simulink model "Main_bikesim2"  (R2024b)
settings: Solver=FixedStepAuto  StartTime=0.0  StopTime=sim_time-0.02  FixedStep=0.005
undefined symbols (not defined in the file): A_d, Ad_t, B_d, Bd_t, bike_model, bike_params, C1, C2, C_t, counter, D1, D2, D_t, e1_max, g, hor_dis, I_balancing_outer, initial_state, initial_state_estimate, k1, k2, Kalman_gain1, Kalman_gain2, linearized_sys, mpc_outer_params, P_balancing_inner, P_balancing_outer, pert_deltadot_state, pert_deltadot_state_fun, pert_phidot_state, pert_phidot_state_fun, Psiref, ref_dis, ref_start_idx, sigbuilder_block, T, Ts, v, Xref, Yref
libraries: simulink x8, slpidlib x2, eeGeneralControl x1
(part 2 of 2)

== matlab function Main_bikesim2/State estimator1/Linearized Bicycle Model on Constant Velocity ==
  data: Est_States input; dot_delta input; y input; Kalman_gain1 input; Kalman_gain2 input; bike_params input; Est_states output; flag input; A_d parameter; B_d parameter; C1 parameter; C2 parameter; D1 parameter; D2 parameter; T parameter
function Est_states  = fcn(Est_States, dot_delta, y, Kalman_gain1, Kalman_gain2, bike_params, flag, A_d, B_d, C1, C2, D1, D2, T)
% description 
% Inputs
%   Est_States := [X Y psi phi phi_dot delta v] are global at time t 
%   dot_delta_e := effective steering rate
%   y := measurement vector
%   Kalman_gain1 := Computed state_feedback gain including GPS meas
%   Kalman_gain2 := Computed state_feedback gain excluding GPS meas
%   bike_params := vector of bike parameters + gravity
%   Ts := Estimator sampling rate
%   v := constant velocity
%   flag := [0-1] increasing counter reseted at 1. When flag == 0 means
%           that GPS measurement is available
%
% Outputs
%   Est_states : = [X Y psi phi phi_dot delta v] global at time t+1


% Transform the states to local frame 
    Est_States_l = zeros(7,1);
    
    Est_States_l(1) = Est_States(1) * cos(Est_States(3)) + Est_States(2) * sin(Est_States(3));
    Est_States_l(2) = -Est_States(1) * sin(Est_States(3)) + Est_States(2) * cos(Est_States(3));
    Est_States_l(3) = 0;        % direction of bike is aligned with X local frame
    Est_States_l(4) = Est_States(4);
    Est_States_l(5) = Est_States(5);
    Est_States_l(6) = Est_States(6);
    Est_States_l(7) = Est_States(7);

% Transform measurements to local frame
    y_l = zeros(size(y));

    y_l(1) = y(1) * cos(Est_States(3)) + y(2) * sin(Est_States(3));
    y_l(2) = -y(1) * sin(Est_States(3)) + y(2) * cos(Est_States(3)); 
    y_l(3) = y(3);
    y_l(4) = y(4);
    y_l(5) = y(5);
    y_l(6) = y(6);
    y_l(7) = y(7);

% Correct for parameter values/sensor positions
% The parameters/positions are measures by us (can differ from true values)
X_gps_mod = bike_params(1);
Y_gps_mod = bike_params(2);
H_gps_mod = bike_params(3);

y_l(1) = y_l(1) - X_gps_mod;
y_l(2) = y_l(2) - Y_gps_mod - H_gps_mod*sin(Est_States(4));

% IMU correction
raw_acc  = [0 y_l(3) 0];
raw_gyro = [y_l(4) 0 y_l(5)];

% Apply the correction to the accelerometer measurement
acc_corr = T*raw_acc';

% Apply the correction to the gyro measurement
gyro_corr = T*raw_gyro';
% Results
y_l(3) =acc_corr(2) ;
y_l(4) =gyro_corr(1) ;
y_l(5) =gyro_corr(3) ;
% 
% % Continuous Time update in local frame TODO: x(t+1) = (I+A delta_T)h_hat(t)
%     states_dot = zeros(7,1);
%     
%     states_dot(1) = Est_States(7);
%     states_dot(2) = v * (Est_States_l(3) + (lr/(lr+lf))*Est_States(6) );
%     states_dot(3) = (v/(lr+lf)) * Est_States(6);
%     states_dot(4) = Est_States(5);
%     states_dot(5) =(g/h)*Est_States(4) + ((lr*v)/((lr+lf)*h))*sin(lambda)*dot_delta + ((h*v^2-g*lr*c)/((lr+lf)*h^2))*sin(lambda)*Est_States(6);
%     states_dot(6) = dot_delta;
%     states_dot(7) = 0;
% 
% % Discrete time update in local 
%     Est_States_l = Est_States_l + states_dot * Ts; 

% % C identity is used to see if the code runs
%     sen = zeros(6,1);
%     sen(1)      = States_l(1);  
%     sen(2)      = States_l(2);
%     %sen(3)      = States_l(3);
%     sen(3)      = States_l(4);
%     sen(4)      = States_l(5);
%     sen(5)      = States_l(6);
%     sen(6)      = States_l(7);

% % Transform measurements into local frame to see if code runs
%     meas_l = zeros(6,1);
%     meas_l(1) = meas(1) * cos(States(3)) + meas(2) * sin(States(3));
%     meas_l(2) = -meas(1) * sin(States(3)) + meas(2) * cos(States(3));
%     meas_l(3) = 0;
%     meas_l(3) = meas(3)-States(3);  
%     meas_l(3) = meas(4);
%     meas_l(4) = meas(5);
%     meas_l(5) = meas(6);
%     meas_l(6) = meas(7);
%     meas_l(7) = meas(7);

% Time update in local frame (from t to t+1)

    % Time update
     Est_States_l = A_d*Est_States_l + B_d*dot_delta;

    % Measurement update in local frame
     Est_states_l = zeros(7,1);

    % Sampling differentiation (Sensors rate 100Hz but GPS 10Hz)

    if flag == 0 % GPS sensors included
    
        % Select Kalman Gain
            K = Kalman_gain1;

        % Measurement prediction
            y_pred = C1*Est_States_l + D1*dot_delta;
    
        % Measurement update
            Est_states_l = Est_States_l + K * (y_l - y_pred);
        
    else % GPS sensors excluded
    
        % Select Kalman Gain
            K = Kalman_gain2;
    
        % Measurement prediction
            y_pred = C2*Est_States_l(4:7) + D2*dot_delta;
 
        % Measurement update
        Est_states_l(1) = Est_States_l(1);
        Est_states_l(2) = Est_States_l(2);
        Est_states_l(3) = Est_States_l(3);
%         Est_states_l(4) = Est_States_l(4);
%         Est_states_l(5) = Est_States_l(5);
%         Est_states_l(6) = Est_States_l(6);
%         Est_states_l(7) = Est_States_l(7);
        Est_states_l(4:7) = Est_States_l(4:7) + K * (y_l(3:7) - y_pred);

    end

    % states_l = Kalman_gain * (meas_l - sen);
    % states_l(1) = States_l(1) + Kalman_gain(1,1) * (meas_l(1) - x_m) + Kalman_gain(1,2) * (meas_l(2) - y_m) + Kalman_gain(1,3) * (meas_l(3) - psi_m) + Kalman_gain(1,4) * (meas_l(4) - phi_m) + Kalman_gain(1,5) * (meas_l(5) - dot_phi_m) + Kalman_gain(1,6) * (meas_l(6) - delta_m) + Kalman_gain(1,7) * (meas_l(7) - v_m);
    % states_l(2) = States_l(2) + Kalman_gain(2,1) * (meas_l(1) - x_m) + Kalman_gain(2,2) * (meas_l(2) - y_m) + Kalman_gain(2,3) * (meas_l(3) - psi_m) + Kalman_gain(2,4) * (meas_l(4) - phi_m) + Kalman_gain(2,5) * (meas_l(5) - dot_phi_m) + Kalman_gain(2,6) * (meas_l(6) - delta_m) + Kalman_gain(2,7) * (meas_l(7) - v_m);
    % states_l(3) = States_l(3) + Kalman_gain(3,1) * (meas_l(1) - x_m) + Kalman_gain(3,2) * (meas_l(2) - y_m) + Kalman_gain(3,3) * (meas_l(3) - psi_m) + Kalman_gain(3,4) * (meas_l(4) - phi_m) + Kalman_gain(3,5) * (meas_l(5) - dot_phi_m) + Kalman_gain(3,6) * (meas_l(6) - delta_m) + Kalman_gain(3,7) * (meas_l(7) - v_m);
    % states_l(4) = States_l(4) + Kalman_gain(4,1) * (meas_l(1) - x_m) + Kalman_gain(4,2) * (meas_l(2) - y_m) + Kalman_gain(4,3) * (meas_l(3) - psi_m) + Kalman_gain(4,4) * (meas_l(4) - phi_m) + Kalman_gain(4,5) * (meas_l(5) - dot_phi_m) + Kalman_gain(4,6) * (meas_l(6) - delta_m) + Kalman_gain(4,7) * (meas_l(7) - v_m);
    % states_l(5) = States_l(5) + Kalman_gain(5,1) * (meas_l(1) - x_m) + Kalman_gain(5,2) * (meas_l(2) - y_m) + Kalman_gain(5,3) * (meas_l(3) - psi_m) + Kalman_gain(5,4) * (meas_l(4) - phi_m) + Kalman_gain(5,5) * (meas_l(5) - dot_phi_m) + Kalman_gain(5,6) * (meas_l(6) - delta_m) + Kalman_gain(5,7) * (meas_l(7) - v_m);
    % states_l(6) = States_l(6) + Kalman_gain(6,1) * (meas_l(1) - x_m) + Kalman_gain(6,2) * (meas_l(2) - y_m) + Kalman_gain(6,3) * (meas_l(3) - psi_m) + Kalman_gain(6,4) * (meas_l(4) - phi_m) + Kalman_gain(6,5) * (meas_l(5) - dot_phi_m) + Kalman_gain(6,6) * (meas_l(6) - delta_m) + Kalman_gain(6,7) * (meas_l(7) - v_m);
    % states_l(7) = States_l(7) + Kalman_gain(7,1) * (meas_l(1) - x_m) + Kalman_gain(7,2) * (meas_l(2) - y_m) + Kalman_gain(7,3) * (meas_l(3) - psi_m) + Kalman_gain(7,4) * (meas_l(4) - phi_m) + Kalman_gain(7,5) * (meas_l(5) - dot_phi_m) + Kalman_gain(7,6) * (meas_l(6) - delta_m) + Kalman_gain(7,7) * (meas_l(7) - v_m);

% Transform to global the local states at time t+1 after measurement update
    Est_states = zeros(7,1);
    Est_states(3) = Est_States(3) + Est_states_l(3);    % direction update global
    
    % Change of Coordinates from local to global frame for  states 
    Est_states(1) = Est_states_l(1) * cos(Est_States(3)) - Est_states_l(2) * sin(Est_States(3));
    Est_states(2) = Est_states_l(1) * sin(Est_States(3)) + Est_states_l(2) * cos(Est_States(3));
    Est_states(4) = Est_states_l(4);
    Est_states(5) = Est_states_l(5);
    Est_states(6) = Est_states_l(6);
    Est_states(7) = Est_states_l(7);
    
    % Heading angle between pi and -pi
    Est_states(3) = wrapToPi(Est_states(3));

end

== matlab function Main_bikesim2/Unstable bike model1/Nonlinear Bicycle model/MATLAB Function ==
  data: States input; xdot output; Steering_rate input; Speed input; disturbances input; bike_params input
function xdot  = fcn(States, Steering_rate, Speed, disturbances, bike_params)
% Unpacked bike_params
    g = bike_params(1);
    h = bike_params(2);
    lr = bike_params(3);
    lf = bike_params(4);
    lambda = bike_params(5);
    c = bike_params(6);
    m = bike_params(7);
    h_imu = bike_params(8);

phi =   States(1);%roll
delta = States(2);%steering angle
phi_d = States(3);%rollrate

% xdot = [phidot deltadot phiddot]
xdot1 = phi_d + disturbances(1);
xdot2 = Steering_rate + disturbances(2);
xdot3 = (g/h)*sin(phi) + ((lr*Speed)/((lr+lf)*h))/(cos(sin(lambda)*delta)^2)*sin(lambda)*Steering_rate ...
                                  + ((Speed^2/h)-(g*lr*c/(h^2*(lr+lf))))*sin(lambda)*tan(delta);

% linearized
% xdot3 = (g/h)*phi + ((lr*Speed)/((lr+lf)*h))*Steering_rate + ((Speed^2/h)-(g*lr*c/(h^2*(lr+lf))))*sin(lambda)*delta;

xdot = [xdot1 xdot2 xdot3]';

== matlab function Main_bikesim2/Unstable bike model1/Track bycicle pose/Derivative of positions ==
  data: Speed input; beta input; psi input; Xdot output; Ydot output
function [Xdot, Ydot]  = fcn(Speed, beta, psi)

Xdot = Speed * cos(psi + beta);
Ydot = Speed * sin(psi + beta);

== matlab function Main_bikesim2/Unstable bike model1/Track bycicle pose/MATLAB Function ==
  data: Speed input; steer_angle input; beta output; bike_params input; psi_dot output
function [beta, psi_dot] = fcn(Speed, steer_angle, bike_params)
lr       = bike_params(1);
lf       = bike_params(2);
lambda  = bike_params(3);

eff_steering = steer_angle*sin(lambda);

beta = atan(lr /(lr+lf) * tan(eff_steering) );
psi_dot = (Speed / lr) * sin(beta);

== matlab function Main_bikesim2/Trajectory controller/Trajectory controller ==
  settings: updateMethod=DISCRETE  sampleTime=Ts
  data: e1 output; e2 output; closestpoint_idx output; closestpoint_heading_idx output; Xref_loc input; Yref_loc input; psiref_loc input; X_est input; Y_est input; psi_est input; bike_params input; v input; h input; ref_X output; ref_Y output; ref_psi output; roll_ref output; delta_ref output; mpc_outer_params parameter; EXITFLAG output; Ad_t parameter; Bd_t parameter; C_t parameter; D_t parameter; h_dot output
function [e1,e2,closestpoint_idx,closestpoint_heading_idx,ref_X,ref_Y,ref_psi,roll_ref,delta_ref,EXITFLAG,h_dot]= fcn(Xref_loc,Yref_loc,psiref_loc,X_est,Y_est,psi_est,bike_params,v, ...
                                                                                                             h, mpc_outer_params, Ad_t, Bd_t, C_t, D_t)
%% calculations on a local part of the trajectory

% Unpack parameters
g  = bike_params(1);
lr = bike_params(2);
lf = bike_params(3);
lambda = bike_params(4);

% Each referencepoint has a location (X,Y) and a heading
% The heading is defined in the startup.m file as 'the heading where its coming from' 
% Second point in local reference is current selected closest point
closestpoint_idx=2;

% Search for closest point
% Finding the closest point going forward. Stop searching once next
% distance increases

while (Xref_loc(closestpoint_idx,1)-X_est)^2 + (Yref_loc(closestpoint_idx,1)-Y_est)^2 >= (Xref_loc(closestpoint_idx+1,1)-X_est)^2+(Yref_loc(closestpoint_idx+1,1)-Y_est)^2  && closestpoint_idx <= length(Xref_loc)-2
closestpoint_idx = closestpoint_idx+1;
end

% Select same closest point (for heading error and position error)
closestpoint_heading_idx = closestpoint_idx;

% Calculate X and Y distance from current location to selected closest
% point
dx = X_est - Xref_loc(closestpoint_idx,1);
dy = Y_est - Yref_loc(closestpoint_idx,1);

% Calculate difference in current heading and heading in reference point 
% And limit D_psiref  between -2pi and 2pi
D_psiref=psiref_loc(closestpoint_idx+1,1)-psiref_loc(closestpoint_idx,1);
if D_psiref>=pi
    D_psiref=mod(D_psiref,-2*pi);
end
if D_psiref<=-pi
    D_psiref=mod(D_psiref,2*pi);
end
if closestpoint_idx > 1
    %IMPROVEMENT: implement an interpolation algoritm
    % Calculate distence between point before closest point and current location
    dist_true_previous = sqrt((Xref_loc(closestpoint_idx-1,1)-X_est)^2+(Yref_loc(closestpoint_idx-1,1)-Y_est)^2);
    % Angle of line between previous closest point and current location
    alpha_star = atan((Yref_loc(closestpoint_idx-1,1)-Y_est)/(Xref_loc(closestpoint_idx-1,1)-X_est));
    % heading previous closest point - alpha star
    alpha_projected_dist = alpha_star-psiref_loc(closestpoint_idx,1);
    % the distance from the previous closest point to the projection of the bike on the trajectory
    Projected_dist = abs(dist_true_previous*cos(alpha_projected_dist));
    
    compared_dist = sqrt((Xref_loc(closestpoint_idx,1)-Xref_loc(closestpoint_idx-1,1))^2+(Yref_loc(closestpoint_idx,1)-Yref_loc(closestpoint_idx-1,1))^2);
    
    % If bike passes closest point, the heading of the next point will be taken
    if Projected_dist >= compared_dist
        closestpoint_heading_idx = closestpoint_idx+1;
    end
end

%calculate e1 and e2        
e1= dy*cos(psiref_loc(closestpoint_heading_idx,1)) - dx*sin(psiref_loc(closestpoint_heading_idx,1)); % this make e1 include "direction" automatically
e2= psi_est-psiref_loc(closestpoint_heading_idx,1); %calculate e2

% closest point on the local trajectory
ref_X=Xref_loc(closestpoint_idx,1);
ref_Y=Yref_loc(closestpoint_idx,1);
ref_psi=psiref_loc(closestpoint_heading_idx,1);

 % keep heading error should be between -pi 2 pi
e2 = wrapToPi(e2);
%e2=mod(e2+pi,2*pi)-pi; 

% MPC controller
A=mpc_outer_params.Ad;
B=mpc_outer_params.Bd;
C=mpc_outer_params.Cd;
D=mpc_outer_params.Dd;
N=mpc_outer_params.N;
Q=mpc_outer_params.Q;
Pf=mpc_outer_params.Pf;
R=mpc_outer_params.R;
F=mpc_outer_params.F;
G=mpc_outer_params.G;
h_mpc=mpc_outer_params.h;

x=[e1 e2]';

%Assemble the Q_bar and R_bar
Q_bar = blkdiag(kron(eye(N-1),Q),Pf);
R_bar = kron(eye(N),R);
%quadratic objective form
H=blkdiag(Q_bar,R_bar);
f=[]; %f is empty due to the lack of linear terms in cost func

%equality constraints
[rowA,colA]=size(A);
[rowB,colB]=size(B);

%Aeq1=zeros(N*rowA,N*colA);
Aeq1=kron(eye(colA),eye(N));

[rowAeq1,colAeq1]=size(Aeq1);

colAeq1Range=[1:colA:colAeq1-colA];
colAeq1Index=1;
% Todo: Replace with kron for speed 
for n=rowA:rowA:rowAeq1-rowA
    Aeq1(n+1:n+rowA,colAeq1Range(colAeq1Index):colAeq1Range(colAeq1Index)+colA-1)=-A;
    colAeq1Index=colAeq1Index+1;
end

Aeq2 = kron(eye(N),-B);

Aeq  = [Aeq1 Aeq2];
beq  = [A*x;zeros(colA*(N-1),1)];

%inequallity
Ain  = [F G];
bin  = h_mpc;

coder.extrinsic('quadprog');
coder.extrinsic('optimset');
% max time tunable...
maxTime=10;
options = optimset('Display', 'off','TolX',1e-2,'TolFun', 1e-3,'MaxTime',maxTime);

EXITFLAG = 0;
[Z,VN,EXITFLAG] = quadprog(2*H,f,Ain,bin,Aeq,beq,[],[],[],options);
delta_ref = 0;
delta_ref=Z(colA*N+1);

D_psiref = psiref_loc(closestpoint_heading_idx+1,1)-psiref_loc(closestpoint_heading_idx,1);
D_psiref = wrapToPi(D_psiref);

%calculate the time between psiref(idx,1) and psiref(idx+1,1)
dX=Xref_loc(closestpoint_heading_idx+1,1)-ref_X;
dY=Yref_loc(closestpoint_heading_idx+1,1)-ref_Y;
dis=sqrt(dX^2+dY^2);
Ts_psi=dis/v;

% Sample dpsiref
dpsiref=(D_psiref)/Ts_psi;

% Steering contribution from heading change
h_dot = Ad_t*h + Bd_t*dpsiref;

delta_ref_psi = (C_t*h + D_t*dpsiref);

% Total steering reference 
%delta_ref = delta_ref_psi + delta_ref;

if delta_ref>=pi/9
    delta_ref=pi/9;
 
end
if delta_ref<=-pi/9
    delta_ref=-pi/9;
end
eff_delta_ref = delta_ref*sin(lambda);
roll_ref = -1*atan((tan(eff_delta_ref)*(v^2/(lr+lf)))/g);
end

== matlab function Main_bikesim2/Selection of local reference from total reference1/Local reference selection & stop funcion ==
  data: last_ids input; ids output; xref input; local_Xref output size=Nn [..30000]; local_Yref output size=Nn [..30000]; local_Psiref output size=Nn [..30000]; yref input; psiref input; closest_point input; ref_dis parameter; hor_dis parameter; stop output; abort input; est input
function [ids,local_Xref,local_Yref,local_Psiref,stop] = fcn(last_ids,xref,yref,psiref,closest_point, ref_dis, hor_dis,abort,est)
% Local reference trajectory starts at point before the current closest
% point and has a length of M

%if closest_point>2
%    ids=last_ids+closest_point-2;      % calculate the initial index of the points that will be sent to next block (first point of local_ref)
%else
%    ids = last_ids;  % Only update if last reference point has been passed
%end

ids = last_ids+closest_point-2;
Ns=ceil(hor_dis/ref_dis);          % Th,Ts is definited in "StudentProject2021.m", Ns is the number of points sent to next block
M=ids+Ns;                          % calculate the end index of the end index that will be sent to next block
n=size(xref,1);                    % size of whole trajectory points 
if M>n                             % if reached near end of reference, local trajectry becomes shorter
    M=n;
end

% Temporary simulation STOP to prevent singularity error once approaching
% the end of the trajectory
% Simulation stops before the end of the reference trajectory
stop = 0;
if ids>=n-ceil(n/20)
    stop = 1;
end


% Start always at second value of total reference
if ids == 1
    ids = 2;
end

% Select local reference from total reference
local_Xref=xref(ids-1:1:M);
local_Yref=yref(ids-1:1:M);
local_Psiref=psiref(ids:1:M);

if(abort)
    [local_Xref,local_Yref,local_Psiref] = genAbortTraj(est(1),est(2),est(3),Ns);
end


end


function [x_ref,y_ref,psi_ref] = genAbortTraj(x_est,y_est,psi_est,N)


step = 0.1; %Step size
r  = 5;
%N = 50;

x_ref = zeros(N,1);
y_ref = zeros(N,1);
psi_ref = zeros(N,1);
x_ref(1) = x_est;
y_ref(1) = y_est;
psi_ref(1) = psi_est;

% CALCULATE CENTER OF CIRCLE 
offset_x = r * sin(-psi_est);
offset_y = r * cos(-psi_est);
x_center = x_est + offset_x;
y_center = y_est + offset_y;

i = 1;
for t = step:step:(N*step-1)
    i = i+1;
    x_ref(i) = r*sin(-t+pi-psi_est) + x_center;
    y_ref(i) = r*cos(-t+pi-psi_est) + y_center;
    psi_ref(i) = atan2(y_ref(i)-y_ref(i-1),x_ref(i)-x_ref(i-1));  
end

end

== matlab function Main_bikesim2/Trajectory controller + closest_point selection/Trajectory controller ==
  settings: updateMethod=DISCRETE  sampleTime=Ts
  data: closestpoint_idx_in input; closestpoint_idx_out output; e1 output; e2 output; closestpoint_heading_idx output; Xref_loc input; Yref_loc input; psiref_loc input; X_est input; Y_est input; psi_est input; bike_params input; traj_error_params input; ref_X output; ref_Y output; ref_psi output; v input; roll_ref output; delta_ref output; delta_e1 output; delta_e2 output; delta_ref_psi output; D_psiref output; x input; x_dot output; Ad_t parameter; Bd_t parameter; C_t parameter; D_t parameter
function [closestpoint_idx_out,e1,e2,closestpoint_heading_idx,ref_X,ref_Y,ref_psi,roll_ref,delta_ref,delta_e1,delta_e2,delta_ref_psi,D_psiref,x_dot]= fcn(closestpoint_idx_in,Xref_loc,Yref_loc,psiref_loc,X_est,Y_est,psi_est,bike_params,traj_error_params, ...
                                                                                                            v, x, Ad_t, Bd_t, C_t, D_t)
%% calculations on a local part of the trajectory

% Unpack parameters
g  = bike_params(1);
lr = bike_params(2);
lf = bike_params(3);
lambda = bike_params(4);

k1 = traj_error_params(1);
k2 = traj_error_params(2);
e1_max = traj_error_params(3);

% Search for closest point --> Finding the closest point going forward. Stop searching once next distance increases
while (Xref_loc(closestpoint_idx_in,1)-X_est)^2 + (Yref_loc(closestpoint_idx_in,1)-Y_est)^2 >= (Xref_loc(closestpoint_idx_in+1,1)-X_est)^2+(Yref_loc(closestpoint_idx_in+1,1)-Y_est)^2  && closestpoint_idx_in <= length(Xref_loc)-2
    closestpoint_idx_in = closestpoint_idx_in+1;
end

% Select same closest point (for heading error and position error)
closestpoint_heading_idx = closestpoint_idx_in;

% Calculate X and Y distance from current location to selected closest
% point
dx = X_est - Xref_loc(closestpoint_idx_in,1);
dy = Y_est - Yref_loc(closestpoint_idx_in,1);

% Calculate difference in current heading and heading in reference point 
% And limit D_psiref  between pi and -pi
D_psiref = psiref_loc(closestpoint_idx_in+1,1)-psiref_loc(closestpoint_idx_in,1);
D_psiref = wrapToPi(D_psiref);
% if D_psiref>=pi
%     D_psiref=mod(D_psiref,-2*pi);
% end
% if D_psiref<=-pi
%     D_psiref=mod(D_psiref,2*pi);
% end

%IMPROVEMENT: implement an interpolation algoritm
% Calculate distence between point before closest point and current location
dist_true_previous = sqrt((Xref_loc(closestpoint_idx_in-1,1)-X_est)^2+(Yref_loc(closestpoint_idx_in-1,1)-Y_est)^2);
% Angle of line between previous closest point and current location
alpha_star = atan((Yref_loc(closestpoint_idx_in-1,1)-Y_est)/(Xref_loc(closestpoint_idx_in-1,1)-X_est));
% heading previous closest point - alpha star
alpha_projected_dist = alpha_star-psiref_loc(closestpoint_idx_in,1);
% the distance from the previous closest point to the projection of the bike on the trajectory
Projected_dist = abs(dist_true_previous*cos(alpha_projected_dist));

compared_dist = sqrt((Xref_loc(closestpoint_idx_in,1)-Xref_loc(closestpoint_idx_in-1,1))^2+(Yref_loc(closestpoint_idx_in,1)-Yref_loc(closestpoint_idx_in-1,1))^2);

% If bike passes closest point, the heading of the next point will be taken
if Projected_dist >= compared_dist
closestpoint_heading_idx = closestpoint_idx_in+1;
end

%calculate e1 and e2        
e1= dy*cos(psiref_loc(closestpoint_heading_idx,1)) - dx*sin(psiref_loc(closestpoint_heading_idx,1)); % this make e1 include "direction" automatically
e2= psi_est-psiref_loc(closestpoint_heading_idx,1); %calculate e2

% closest point on the local trajectory
ref_X=Xref_loc(closestpoint_idx_in,1);
ref_Y=Yref_loc(closestpoint_idx_in,1);
ref_psi=psiref_loc(closestpoint_heading_idx,1);

 % keep heading error should be between -pi 2 pi
e2 = wrapToPi(e2);
%e2=mod(e2+pi,2*pi)-pi;     

%calculate the time between psiref(idx,1) and psiref(idx+1,1)
dX=Xref_loc(closestpoint_idx_in+1,1)-ref_X;
dY=Yref_loc(closestpoint_idx_in+1,1)-ref_Y;
dis=sqrt(dX^2+dY^2);
Ts_psi=dis/v;

% Sample dpsiref
dpsiref=(D_psiref)/Ts_psi;

% Loop the closest point
closestpoint_idx_out = closestpoint_idx_in;

% Steering contribution from trajectory error
% delta_ref_error=-k1*sign(e1)*min(abs(e1),e1_max)-k2*e2;
delta_e1 = -k1*sign(e1)*min(abs(e1),e1_max);
delta_e2 =-k2*e2;
% delta_e1 = -2;
% delta_e2 = 0;
delta_ref_error = delta_e1 + delta_e2;

% Steering contribution from heading change
x_dot = Ad_t*x + Bd_t*dpsiref;
delta_ref_psi = (C_t*x + D_t*dpsiref); 
% delta_ref_psi = 0; 

% Total steering reference 
delta_ref = delta_ref_psi + delta_ref_error;

% limit steer angle between -pi/4 and pi/4
if delta_ref>=pi/4
    delta_ref=pi/4;
end

if delta_ref<=-pi/4
    delta_ref=-pi/4;
end

% Transform steering reference into roll reference for balancing controller
eff_delta_ref = delta_ref*sin(lambda);
roll_ref = -1*atan(tan(eff_delta_ref)*(v^2/(lr+lf))/g);

end
